simulink model "hnn_matrix"  (R2024b)
settings: Solver=VariableStepAuto  StartTime=0.0  StopTime=10.0  RelTol=1e-3
settings Model: Creator=merlin  LastModifiedBy=merlin

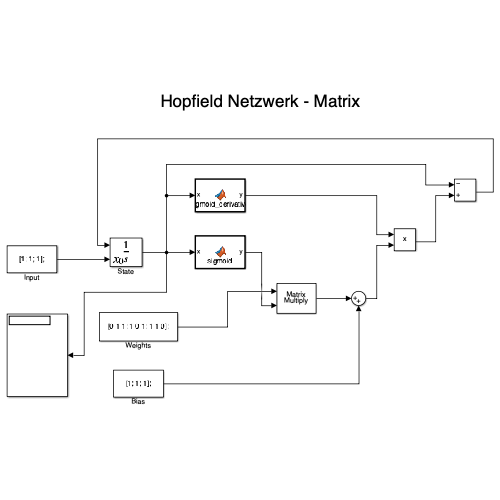
[thumbnail: Simulink's stored preview of the top-level diagram]
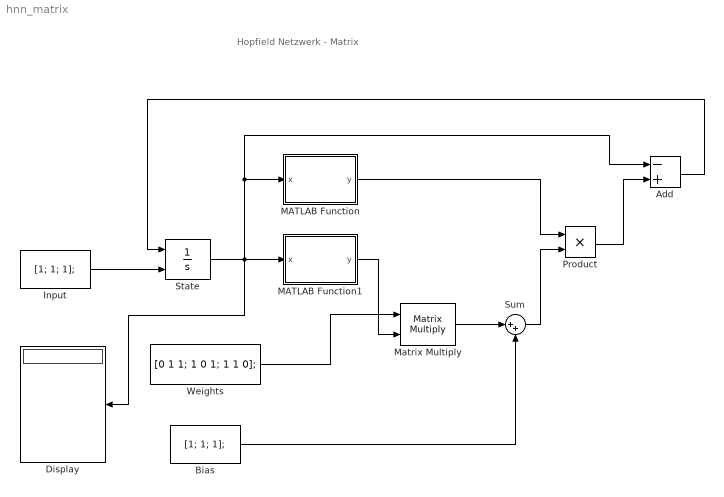
== system hnn_matrix ==
  note: Hopfield Netzwerk - Matrix
  Add : Sum  Inputs=-+
  Bias : Constant  Value=[1; 1; 1];  VectorParams1D=off
  Display : Display
  Input : Constant  Value=[1; 1; 1];  VectorParams1D=off
  MATLAB Function : MATLAB Function  TreatAsAtomicUnit=on
  MATLAB Function1 : MATLAB Function  TreatAsAtomicUnit=on
  Matrix Multiply : Product  Multiplication=Matrix(*)
  Product : Product
  State : Integrator  InitialConditionSource=external
  Sum : Sum  Inputs=|++
  Weights : Constant  Value=[0 1 1; 1 0 1; 1 1 0];  VectorParams1D=off
  wires:
  MATLAB Function/1(y) -> Product/1
  Product/1 -> Add/2
  Sum/1 -> Product/2
  State/1 -> MATLAB Function/1(x), Add/1, Display/1, MATLAB Function1/1(x)
  Bias/1 -> Sum/2
  Weights/1 -> Matrix Multiply/1
  Input/1 -> State/2
  MATLAB Function1/1(y) -> Matrix Multiply/2
  Matrix Multiply/1 -> Sum/1
  Add/1 -> State/1

== matlab function hnn_matrix/MATLAB Function ==
  data: x input; y output
function y = sigmoid_derivative(x)
sigmoid = 1 ./ (1 + exp(-x));
y = sigmoid .* (1 - sigmoid);
end

== matlab function hnn_matrix/MATLAB Function1 ==
  data: x input; y output
function y = sigmoid(x)
y = 1 ./ (1 + exp(-x));
end
